simulink model "Prototype7C"  (R2015a)
settings: Solver=ode45  SolverMode=SingleTasking  StartTime=0.0  StopTime=17.0  RelTol=1e-3
PreLoadFcn:
  | load 'RegionInterest.mat'
undefined symbols (not defined in the file): gray, HDTV, Rec, RegionOfInterestLane
libraries: visiontransforms x2, visionanalysis x2, dspvision x1, visionstatistics x1, visiontextngfix x1, dspadpt3 x1, visionsinks x1, visionconversions x1
settings Model: Creator=Andrew H  LastModifiedBy=Andrew H
settings OptimizationCC: BlockReduction=off  BooleanDataType=off
settings DebuggingCC: SaveWithParameterizedLinksMsg=none  UnderspecifiedInitializationDetection=Classic  MergeDetectMultiDrivingBlocksExec=none  SignalResolutionControl=TryResolveAllWithWarning
settings HardwareCC: TargetUnknown=on

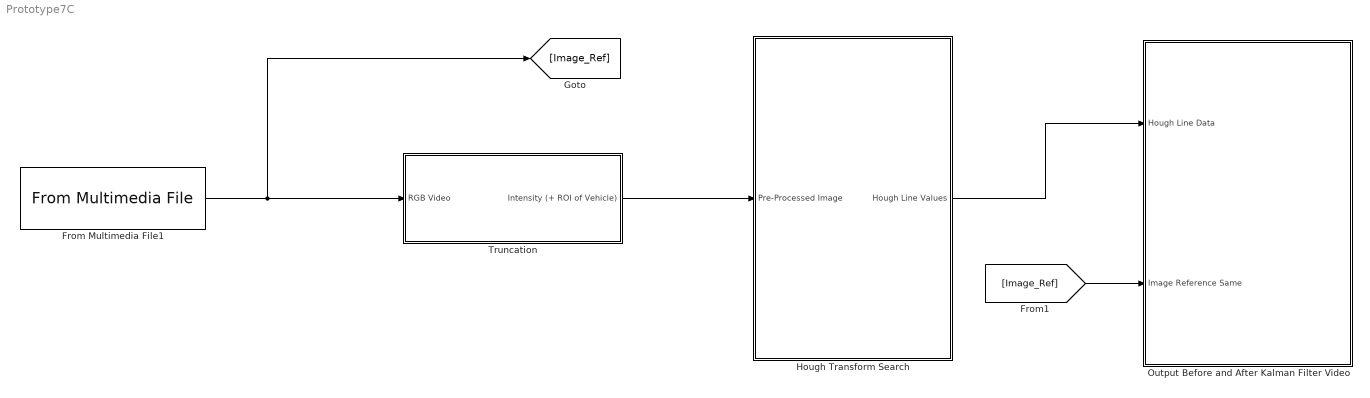
== system Prototype7C ==
  From Multimedia File1 : dspvision/From Multimedia File  inputFilename=C:\Users\Andrew H\Desktop\Video.mp4  loop=on  numPlays=inf  outputStreams=Video only  videoDataType=single  audioDataType=int16  inheritSampleTime=on  userDefinedSampleTime=1/30  noAudioOutput=off  isIntensityVideo=off  fourcc=RGB  colorVideoFormat=One multidimensional signal  outputEOF=off  dataOrg=Column-major  audioFrameSize=1024  computeAudioFrameSize=off  outSamplingMode=Sample based
  Hough Transform Search : Subsystem
  Output Before and After Kalman Filter Video : Subsystem
  Truncation : Subsystem
  wires:
  From Multimedia File1/1 -> [Image_Ref], Truncation/1(RGB Video)
  Truncation/1(Intensity (+ ROI of Vehicle)) -> Hough Transform Search/1(Pre-Processed Image)
  Hough Transform Search/1(Hough Line Values) -> Output Before and After Kalman Filter Video/1(Hough Line Data)
  [Image_Ref] -> Output Before and After Kalman Filter Video/2(Image Reference Same)

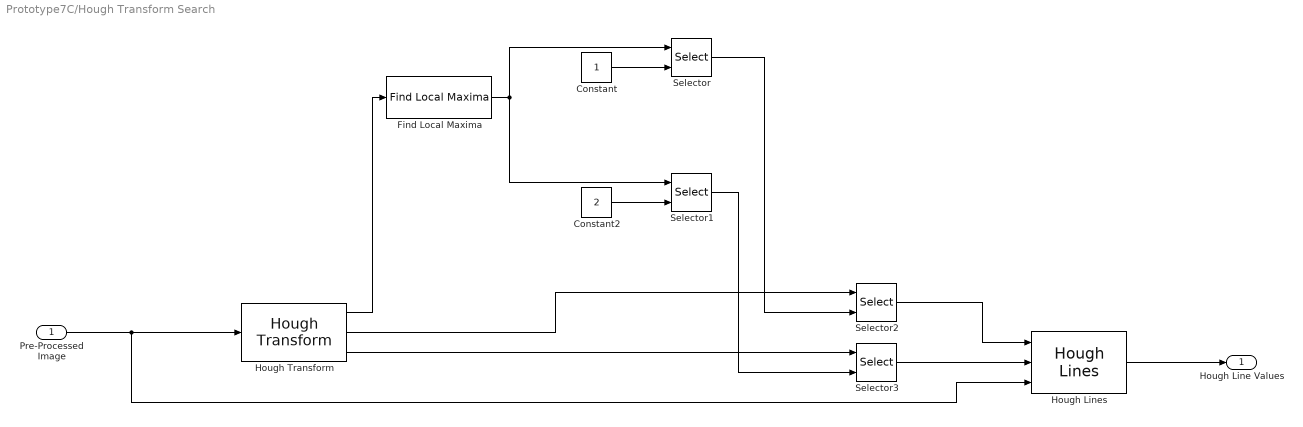
== system Prototype7C/Hough Transform Search ==
  Pre-Processed Image : Inport
  Constant : Constant
  Constant2 : Constant  Value=2
  Find Local Maxima : visionstatistics/Find Local Maxima  num_peaks=1  nhood_size=[5 7]  src_thresh=Obsolete9b  src_thresh_inuse=Specify via dialog  threshold=10  inputIsHough=on  dt_peak=uint32  isOutVarDim=on  dt_count=uint32
  Hough Lines : visiontransforms/Hough Lines  sineCompMethod=Trigonometric function  thetaRes=pi/180  firstCoeffMode=Specify word length  firstCoeffWordLength=16  firstCoeffFracLength=15  prodOutputMode=Binary point scaling  prodOutputWordLength=32  prodOutputFracLength=16  roundingMode=Nearest  overflowMode=on
  Hough Transform : visiontransforms/Hough Transform  theta_res=pi/180  rho_res=1  out_theta_rho=on  outdtmode=double  firstCoeffMode=Binary point scaling  firstCoeffWordLength=16  firstCoeffFracLength=14  secondCoeffMode=Binary point scaling  secondCoeffWordLength=32  secondCoeffFracLength=16  outputMode=Binary point scaling  outputWordLength=16  outputFracLength=0  accumMode=Binary point scaling  accumWordLength=32  accumFracLength=20  prodOutputMode=Binary point scaling  prodOutputWordLength=32  prodOutputFracLength=20  memoryMode=Binary point scaling  memoryWordLength=32  memoryFracLength=16  roundingMode=Nearest  overflowMode=on
  Selector : Selector  InputPortWidth=2  IndexOptions=Index vector (port)
  Selector1 : Selector  InputPortWidth=2  IndexOptions=Index vector (port)
  Selector2 : Selector  NumberOfDimensions=2  InputPortWidth=2  IndexOptions=Select all,Index vector (port)  Indices=1,1  OutputSizes=1,1
  Selector3 : Selector  NumberOfDimensions=2  InputPortWidth=2  IndexOptions=Select all,Index vector (port)  Indices=1,1  OutputSizes=1,1
  Hough Line Values : Outport
  wires:
  Hough Lines/1 -> Hough Line Values/1
  Selector1/1 -> Selector3/2
  Constant2/1 -> Selector1/2
  Selector2/1 -> Hough Lines/1
  Hough Transform/1 -> Find Local Maxima/1
  Selector3/1 -> Hough Lines/2
  Hough Transform/3 -> Selector3/1
  Constant/1 -> Selector/2
  Selector/1 -> Selector2/2
  Pre-Processed Image/1 -> Hough Transform/1, Hough Lines/3
  Find Local Maxima/1 -> Selector/1, Selector1/1
  Hough Transform/2 -> Selector2/1

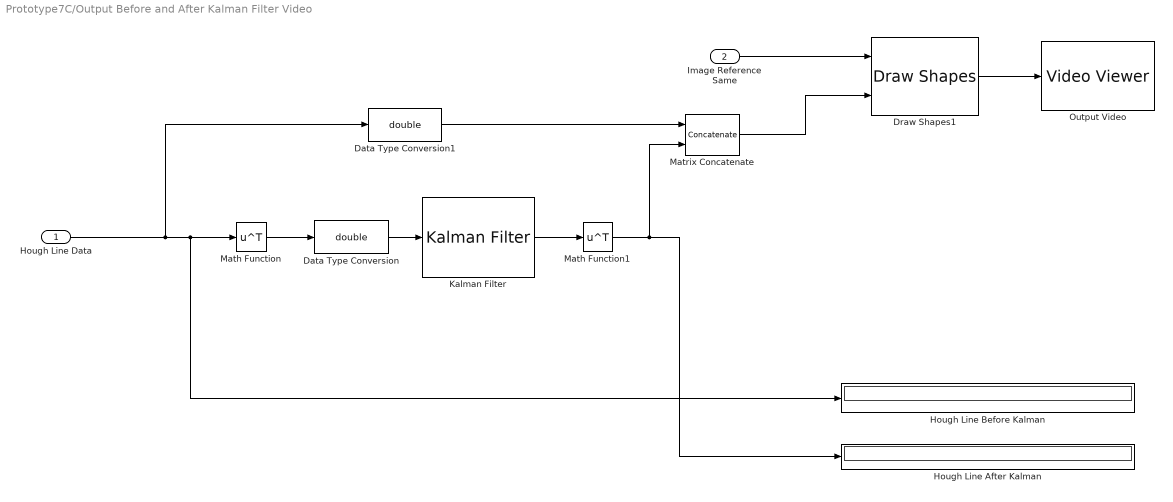
== system Prototype7C/Output Before and After Kalman Filter Video ==
  Hough Line Data : Inport
  Image Reference Same : Inport  Port=2
  Data Type Conversion : DataTypeConversion  OutDataTypeStr=double
  Data Type Conversion1 : DataTypeConversion  OutDataTypeStr=double
  Draw Shapes1 : visiontextngfix/Draw Shapes  shape=Lines  fill=off  lineWidth=4  fillClrSource=Specify via dialog  display=User-specified value  intensity=200  color=[0 0 255; 255 0 0]  opacity=0.6  viewport=Entire image  antialiasing=off  inType=Obsolete  imagePorts=One multidimensional signal  prodOutputMode=Binary point scaling  prodOutputWordLength=32  prodOutputFracLength=14  memoryMode=Specify word length  memoryWordLength=16  memoryFracLength=14  roundingMode=Floor  overflowMode=off
  Hough Line After Kalman : Display
      settings: Decimation=2
  Hough Line Before Kalman : Display
      settings: Decimation=2
  Kalman Filter : dspadpt3/Kalman Filter  num_targets=1  sourceEnable=Always  isReset=on  X=zeros([4, 1])  P=10*eye(4)  A=[1 0 0 0; 0 1 0 0; 0 0 1 0;0 0 0 1]  sourceMeasure=Specify via Dialog  H=[1 0 0 0; 0 1 0 0; 0 0 1 0; 0 0 0 1]  Q=0.05*eye(4)  R=eye(4)  isOutputEstMeasure=on  isOutputEstState=off  isOutputEstError=off  isOutputPrdMeasure=off  isOutputPrdState=off  isOutputPrdError=off
  Math Function : Math  Operator=transpose  SaturateOnIntegerOverflow=on
  Math Function1 : Math  Operator=transpose  SaturateOnIntegerOverflow=on
  Matrix Concatenate : Concatenate  Mode=Multidimensional array
  Output Video : visionsinks/Video Viewer  inputType=Obsolete7b  imagePorts=One multidimensional signal  useColorMap=off  colormapValue=gray(256)  specRange=off  minInputVal=0  maxInputVal=255  FigPos=[1 1038 1920 938]  AxisZoom=on  trueSizedOnce=off  OpenAtMdlStart=on  DefaultConfigurationName=vipscopes.VideoViewerScopeCfg
  wires:
  Kalman Filter/1 -> Math Function1/1
  Draw Shapes1/1 -> Output Video/1
  Math Function/1 -> Data Type Conversion/1
  Data Type Conversion/1 -> Kalman Filter/1
  Hough Line Data/1 -> Data Type Conversion1/1, Hough Line Before Kalman/1, Math Function/1
  Image Reference Same/1 -> Draw Shapes1/1
  Matrix Concatenate/1 -> Draw Shapes1/2
  Math Function1/1 -> Hough Line After Kalman/1, Matrix Concatenate/2
  Data Type Conversion1/1 -> Matrix Concatenate/1

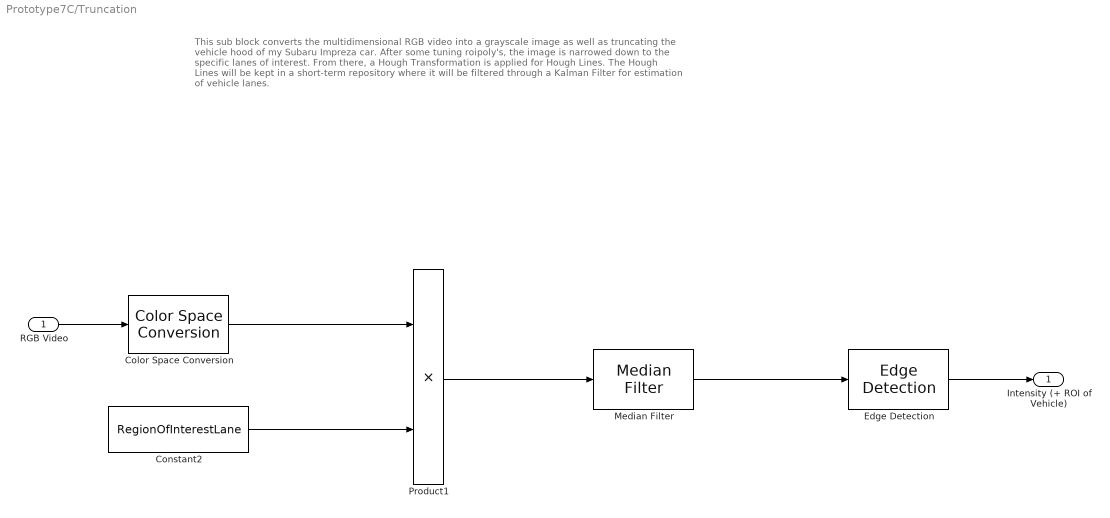
== system Prototype7C/Truncation ==
  note: This sub block converts the multidimensional RGB video into a grayscale image as well
      | as truncating the vehicle hood of my Subaru Impreza car. After some tuning roipoly's, the image is narrowed down to the specific lanes of interest. From there, a Hough Transformation is applied for Hough Lines. The Hough Lines will be kept in a short-term repository where it will be filtered through a Kalman Filter for estimation of vehicle lanes.
  RGB Video : Inport
  Color Space Conversion : visionconversions/Color Space  Conversion  conversion=Obsolete  conversionActive=R'G'B' to intensity  wp_str=D65  rec=Rec. 709 (HDTV)  sys=1125/60/2:1  imagePorts=One multidimensional signal
  Constant2 : Constant  Value=RegionOfInterestLane
  Edge Detection : visionanalysis/Edge Detection  method=Sobel  outputType=Binary image  userDefinedThreshold=off  thresholdSource=Input port  threshold=20  thresholdTuning=4  edgeThinning=off  threshold_canny=[0.25 0.60]  autoPercent=70  sigma=1  prodOutputMode=Binary point scaling  prodOutputWordLength=32  prodOutputFracLength=8  roundingMode=Floor  overflowMode=off
  Median Filter : visionanalysis/Median Filter  nghbood=[5 5]  outSize=Same as input port I  padType=Symmetric  padSrc=Specify via dialog  padVal=0  roundingMode=Floor  overflowMode=off
  Product1 : Product
  Intensity (+ ROI of Vehicle) : Outport
  wires:
  Color Space Conversion/1 -> Product1/1
  Product1/1 -> Median Filter/1
  Median Filter/1 -> Edge Detection/1
  Edge Detection/1 -> Intensity (+ ROI of Vehicle)/1
  Constant2/1 -> Product1/2
  RGB Video/1 -> Color Space Conversion/1
